simulink model "sm_five_bar_robot_control"  (R2021b)
settings: Solver=ode15s  StartTime=0.0  StopTime=tt(end)  FixedStep=0.0001  RelTol=1e-3  AbsTol=1e-3  EnableMultiTasking=on
model workspace: external: MATLAB File sm_five_bar_robot_parameters.m (data not in the file)
undefined symbols (not defined in the file): dT_target, Fq_interp, Kd, Kd_joint1_1, Ki, Ki_joint1_1, Kp, Kp_2, l0, m1, m2, m_gripper, N, N_joint1_1, Q_interp, Qp_interp, Qpp_interp, smiData, X, Y, Z
libraries: sm_lib x44, nesl_utility x25, slpidlib x4
(part 3 of 3)

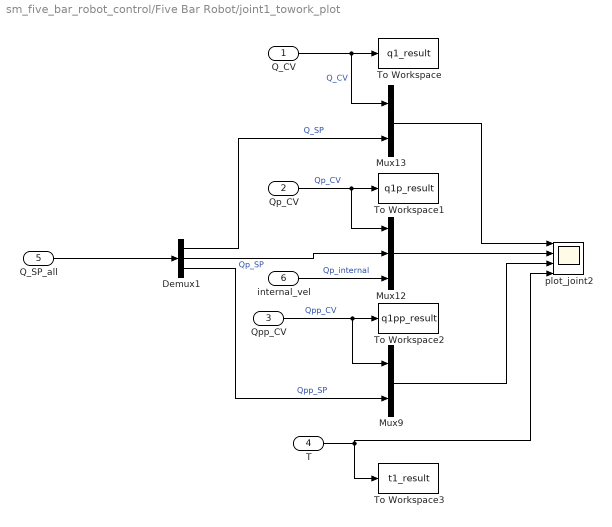
== system sm_five_bar_robot_control/Five Bar Robot/joint1_towork_plot ==
  Q_CV : Inport
  Qp_CV : Inport  Port=2
  Qpp_CV : Inport  Port=3
  T : Inport  Port=4
  Q_SP_all : Inport  Port=5
  internal_vel : Inport  Port=6
  Demux1 : Demux  Outputs=3
  Mux12 : Mux  Inputs=3
  Mux13 : Mux  Inputs=2
  Mux9 : Mux  Inputs=2
  To Workspace : ToWorkspace  VariableName=q1_result  SaveFormat=Timeseries  SampleTime=-1
  To Workspace1 : ToWorkspace  VariableName=q1p_result  SaveFormat=Timeseries  SampleTime=-1
  To Workspace2 : ToWorkspace  VariableName=q1pp_result  SaveFormat=Timeseries  SampleTime=-1
  To Workspace3 : ToWorkspace  VariableName=t1_result  SaveFormat=Structure With Time  SampleTime=-1
  plot_joint2 : Scope  NumInputPorts=4
  wires:
  Demux1/1 -> Mux13/2  "Q_SP"
  Demux1/2 -> Mux12/2  "Qp_SP"
  Qpp_CV/1 -> Mux9/1, To Workspace2/1  "Qpp_CV"
  Qp_CV/1 -> Mux12/1, To Workspace1/1  "Qp_CV"
  Q_CV/1 -> Mux13/1, To Workspace/1  "Q_CV"
  T/1 -> plot_joint2/4, To Workspace3/1
  Demux1/3 -> Mux9/2  "Qpp_SP"
  Q_SP_all/1 -> Demux1/1
  Mux13/1 -> plot_joint2/1
  Mux12/1 -> plot_joint2/2
  Mux9/1 -> plot_joint2/3
  internal_vel/1 -> Mux12/3  "Qp_internal"

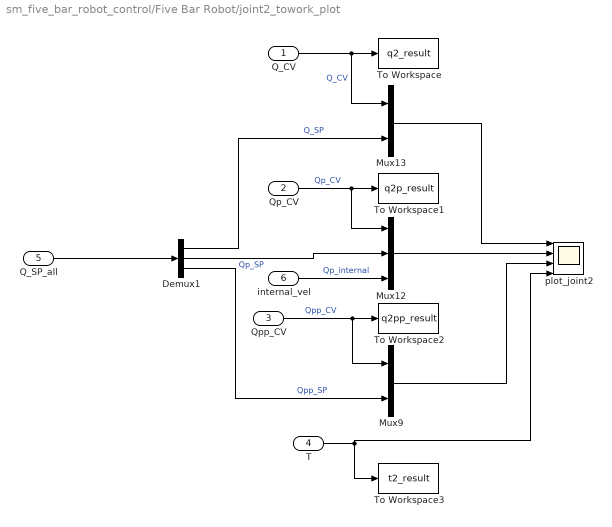
== system sm_five_bar_robot_control/Five Bar Robot/joint2_towork_plot ==
  Q_CV : Inport
  Qp_CV : Inport  Port=2
  Qpp_CV : Inport  Port=3
  T : Inport  Port=4
  Q_SP_all : Inport  Port=5
  internal_vel : Inport  Port=6
  Demux1 : Demux  Outputs=3
  Mux12 : Mux  Inputs=3
  Mux13 : Mux  Inputs=2
  Mux9 : Mux  Inputs=2
  To Workspace : ToWorkspace  VariableName=q2_result  SaveFormat=Timeseries  SampleTime=-1
  To Workspace1 : ToWorkspace  VariableName=q2p_result  SaveFormat=Timeseries  SampleTime=-1
  To Workspace2 : ToWorkspace  VariableName=q2pp_result  SaveFormat=Timeseries  SampleTime=-1
  To Workspace3 : ToWorkspace  VariableName=t2_result  SaveFormat=Structure With Time  SampleTime=-1
  plot_joint2 : Scope  NumInputPorts=4
  wires:
  Demux1/1 -> Mux13/2  "Q_SP"
  Demux1/2 -> Mux12/2  "Qp_SP"
  Qpp_CV/1 -> Mux9/1, To Workspace2/1  "Qpp_CV"
  Qp_CV/1 -> Mux12/1, To Workspace1/1  "Qp_CV"
  Q_CV/1 -> Mux13/1, To Workspace/1  "Q_CV"
  T/1 -> plot_joint2/4, To Workspace3/1
  Demux1/3 -> Mux9/2  "Qpp_SP"
  Q_SP_all/1 -> Demux1/1
  Mux13/1 -> plot_joint2/1
  Mux12/1 -> plot_joint2/2
  Mux9/1 -> plot_joint2/3
  internal_vel/1 -> Mux12/3  "Qp_internal"

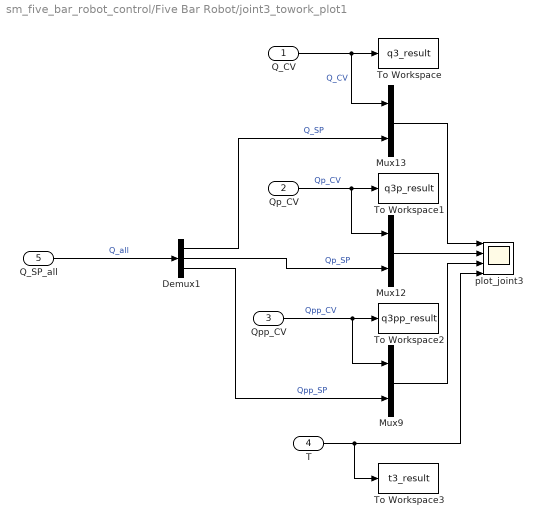
== system sm_five_bar_robot_control/Five Bar Robot/joint3_towork_plot1 ==
  Q_CV : Inport
  Qp_CV : Inport  Port=2
  Qpp_CV : Inport  Port=3
  T : Inport  Port=4
  Q_SP_all : Inport  Port=5
  Demux1 : Demux  Outputs=3
  Mux12 : Mux  Inputs=2
  Mux13 : Mux  Inputs=2
  Mux9 : Mux  Inputs=2
  To Workspace : ToWorkspace  VariableName=q3_result  SaveFormat=Structure With Time  SampleTime=-1
  To Workspace1 : ToWorkspace  VariableName=q3p_result  SaveFormat=Structure With Time  SampleTime=-1
  To Workspace2 : ToWorkspace  VariableName=q3pp_result  SaveFormat=Structure With Time  SampleTime=-1
  To Workspace3 : ToWorkspace  VariableName=t3_result  SaveFormat=Structure With Time  SampleTime=-1
  plot_joint3 : Scope  NumInputPorts=4
  wires:
  Mux9/1 -> plot_joint3/3
  Demux1/1 -> Mux13/2  "Q_SP"
  Mux13/1 -> plot_joint3/1
  Mux12/1 -> plot_joint3/2
  Demux1/2 -> Mux12/2  "Qp_SP"
  Qpp_CV/1 -> Mux9/1, To Workspace2/1  "Qpp_CV"
  Qp_CV/1 -> Mux12/1, To Workspace1/1  "Qp_CV"
  Q_CV/1 -> Mux13/1, To Workspace/1  "Q_CV"
  T/1 -> To Workspace3/1, plot_joint3/4
  Demux1/3 -> Mux9/2  "Qpp_SP"
  Q_SP_all/1 -> Demux1/1  "Q_all"

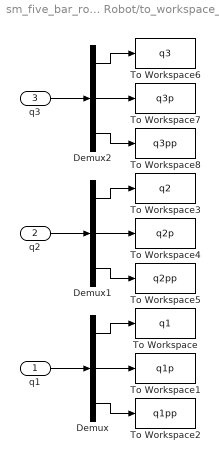
== system sm_five_bar_robot_control/Five Bar Robot/to_workspace_q ==
  q1 : Inport
  q2 : Inport  Port=2
  q3 : Inport  Port=3
  Demux : Demux  Outputs=3
  Demux1 : Demux  Outputs=3
  Demux2 : Demux  Outputs=3
  To Workspace : ToWorkspace  VariableName=q1  SaveFormat=Structure With Time  SampleTime=-1
  To Workspace1 : ToWorkspace  VariableName=q1p  SaveFormat=Structure With Time  SampleTime=-1
  To Workspace2 : ToWorkspace  VariableName=q1pp  SaveFormat=Structure With Time  SampleTime=-1
  To Workspace3 : ToWorkspace  VariableName=q2  SaveFormat=Structure With Time  SampleTime=-1
  To Workspace4 : ToWorkspace  VariableName=q2p  SaveFormat=Structure With Time  SampleTime=-1
  To Workspace5 : ToWorkspace  VariableName=q2pp  SaveFormat=Structure With Time  SampleTime=-1
  To Workspace6 : ToWorkspace  VariableName=q3  SaveFormat=Structure With Time  SampleTime=-1
  To Workspace7 : ToWorkspace  VariableName=q3p  SaveFormat=Structure With Time  SampleTime=-1
  To Workspace8 : ToWorkspace  VariableName=q3pp  SaveFormat=Structure With Time  SampleTime=-1
  wires:
  Demux/1 -> To Workspace/1
  Demux1/1 -> To Workspace3/1
  Demux/2 -> To Workspace1/1
  Demux1/2 -> To Workspace4/1
  Demux/3 -> To Workspace2/1
  Demux1/3 -> To Workspace5/1
  q1/1 -> Demux/1
  q2/1 -> Demux1/1
  q3/1 -> Demux2/1
  Demux2/1 -> To Workspace6/1
  Demux2/2 -> To Workspace7/1
  Demux2/3 -> To Workspace8/1

== matlab function sm_five_bar_robot_control/Five Bar Robot/Trajectory Generator ==
  data: t input; dT_target parameter; q1 output; q1p output; q1pp output; q2 output; q2p output; q2pp output; q3 output; q3p output; q3pp output; Q_interp parameter; Qp_interp parameter; Qpp_interp parameter; Fq1 output; Fq2 output; Fq3 output; Fq_interp parameter
function [q1, q1p,q1pp,q2,q2p,q2pp,q3,q3p,q3pp,Fq1,Fq2,Fq3] = traj_gen(t,dT_target, ...
                                    Q_interp,Qp_interp,Qpp_interp,Fq_interp)

                                
    val=find(dT_target<=t);
    indice=val(end);                         
    
    q1 = Q_interp(indice,1);
    q2 = Q_interp(indice,2);
    q3 = Q_interp(indice,3);
    q1p = Qp_interp(indice,1);
    q2p = Qp_interp(indice,2);
    q3p = Qp_interp(indice,3);
    q1pp = Qpp_interp(indice,1);
    q2pp = Qpp_interp(indice,2);
    q3pp = Qpp_interp(indice,3);
    Fq1=0;
    Fq2=0;
    Fq3=0;

  
end
